simulink model "coordinate_transform_test"  (R2019a)
settings: Solver=VariableStepAuto  StartTime=0.0  StopTime=10.0  RelTol=1e-3
PreLoadFcn:
  | Xscale=1;
  | Yscale=1;
settings Model: Creator=The MathWorks, Inc.  LastModifiedBy=sjayagop
settings DataIOCC: SaveOutput=off  ReturnWorkspaceOutputs=off
settings DebuggingCC: RootOutportRequireBusObject=none  ArithmeticOperatorsInVariantConditions=warning

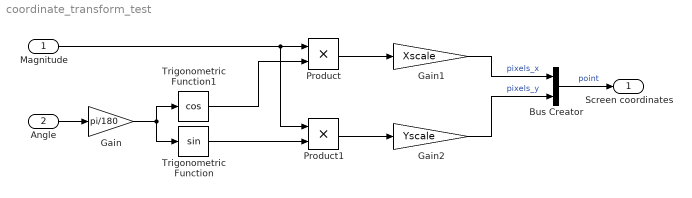
== system coordinate_transform_test ==
  Magnitude : Inport
  Angle : Inport  Port=2
  Bus Creator : BusCreator  Inputs=2
  Gain : Gain  Gain=pi/180
  Gain1 : Gain  Gain=Xscale
  Gain2 : Gain  Gain=Yscale
  Product : Product
  Product1 : Product
  Trigonometric Function : Trigonometry
  Trigonometric Function1 : Trigonometry  Operator=cos
  Screen coordinates : Outport
  wires:
  Angle/1 -> Gain/1
  Gain/1 -> Trigonometric Function1/1, Trigonometric Function/1
  Magnitude/1 -> Product1/1, Product/1
  Trigonometric Function1/1 -> Product/2
  Trigonometric Function/1 -> Product1/2
  Product/1 -> Gain1/1
  Product1/1 -> Gain2/1
  Gain1/1 -> Bus Creator/1  "pixels_x"
  Gain2/1 -> Bus Creator/2  "pixels_y"
  Bus Creator/1 -> Screen coordinates/1  "point"
